simulink model "mMultiTorsionalCompliance"  (R2019b)
settings: Solver=ode4  StartTime=0.0  StopTime=1  FixedStep=.001  RelTol=1e-3
undefined symbols (not defined in the file): DiffAxleDamping, DiffAxleStiffness, DiffDriveshaftDamping, DiffDriveshaftStiffness
libraries: autolibsharedcoupling x6, autolibshareddiff x3, autolibpowerinfoutils x2, VsrLibCoupling x1
settings Model: Creator=9bt  LastModifiedBy=4qz

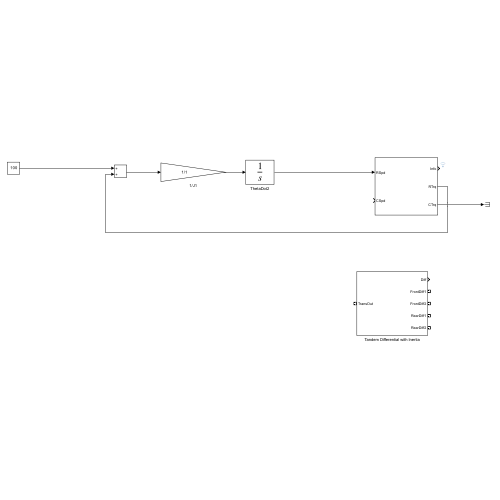
[thumbnail: Simulink's stored preview of the top-level diagram]
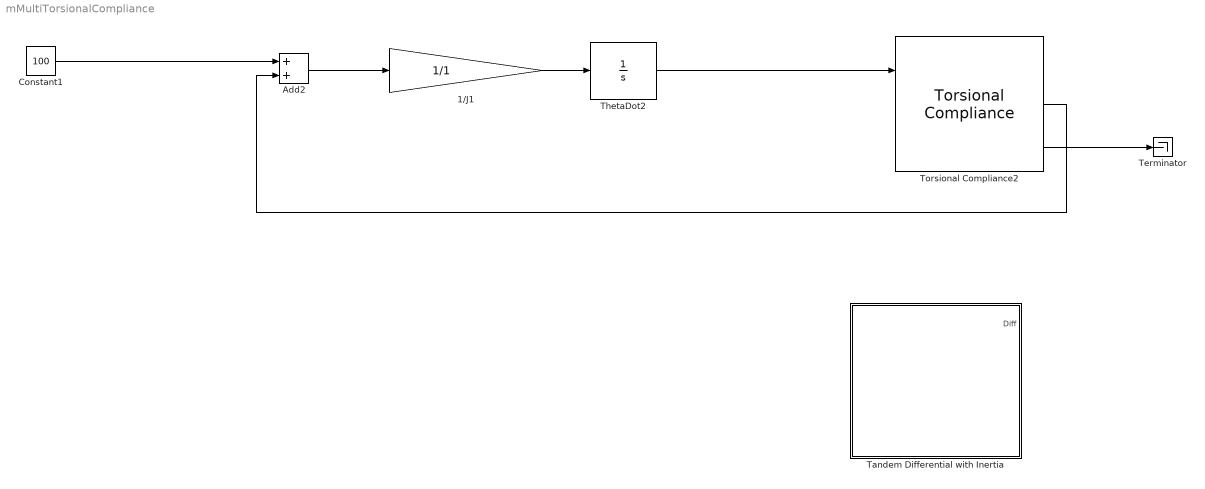
== system mMultiTorsionalCompliance ==
  1/J1 : Gain  Gain=1/1
  Add2 : Sum
  Constant1 : Constant  Value=100
  Tandem Differential with Inertia : Subsystem
  Terminator : Terminator
  ThetaDot2 : Integrator
  Torsional Compliance2 : VsrLibCoupling/Torsional Compliance  StiffnessCalcMethodPopup=Shaft dimensions and material properties  DampingCalcMethodPopup=Damping ratio  D_o=.066  D_i=0  L_shaft=.05  G=77e9  Jcalc=1  zeta=.5  wn=1693.7456  wd=1466.8267  k=2868774.14  b=1197.659  omega_c=500  theta_0=0  omega_0=0
  wires:
  ThetaDot2/1 -> Torsional Compliance2/1
  Add2/1 -> 1/J1/1
  Constant1/1 -> Add2/1
  1/J1/1 -> ThetaDot2/1
  Torsional Compliance2/2 -> Add2/2
  Torsional Compliance2/3 -> Terminator/1

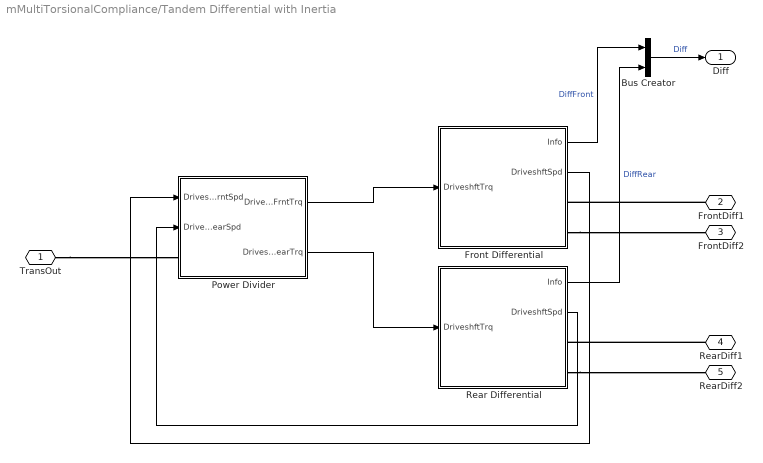
== system mMultiTorsionalCompliance/Tandem Differential with Inertia ==
  Bus Creator : BusCreator  Inputs=2
  Front Differential : Subsystem
  Power Divider : Subsystem
  Rear Differential : Subsystem
  TransOut : PMIOPort  Side=Left
  FrontDiff1 : PMIOPort  Port=2  Side=Right
  FrontDiff2 : PMIOPort  Port=3  Side=Right
  RearDiff1 : PMIOPort  Port=4  Side=Right
  RearDiff2 : PMIOPort  Port=5  Side=Right
  Diff : Outport
  wires:
  Front Differential/1(Info) -> Bus Creator/1  "DiffFront"
  Rear Differential/1(Info) -> Bus Creator/2  "DiffRear"
  Power Divider/2(DriveshftRearTrq) -> Rear Differential/1(DriveshftTrq)
  Power Divider/1(DriveshftFrntTrq) -> Front Differential/1(DriveshftTrq)
  Front Differential/2(DriveshftSpd) -> Power Divider/1(DriveshftFrntSpd)
  Bus Creator/1 -> Diff/1  "Diff"
  Rear Differential/2(DriveshftSpd) -> Power Divider/2(DriveshftRearSpd)
  connections:
  Rear Differential/RConn2 -- RearDiff2/RConn1
  RearDiff1/RConn1 -- Rear Differential/RConn1
  Front Differential/RConn2 -- FrontDiff2/RConn1
  TransOut/RConn1 -- Power Divider/LConn1
  FrontDiff1/RConn1 -- Front Differential/RConn1

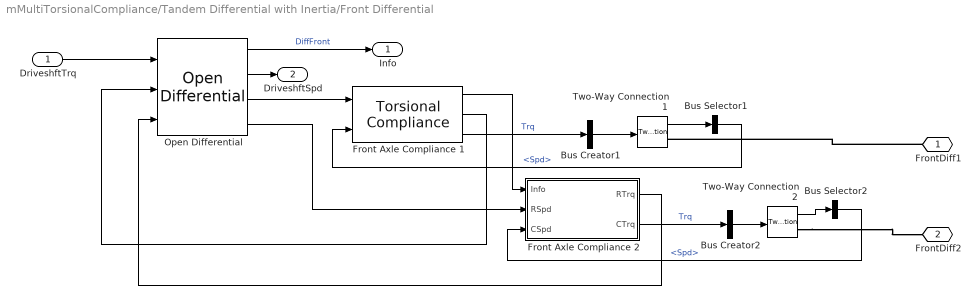
== system mMultiTorsionalCompliance/Tandem Differential with Inertia/Front Differential ==
  DriveshftTrq : Inport
  Bus Creator1 : BusCreator  Inputs=1
  Bus Creator2 : BusCreator  Inputs=1
  Bus Selector1 : BusSelector  OutputSignals=Spd
  Bus Selector2 : BusSelector  OutputSignals=Spd
  Front Axle Compliance 1 : autolibsharedcoupling/Torsional Compliance  port_config=Simulink  extInfo=on  k=DiffAxleStiffness  b=DiffAxleDamping  theta_o=0  domega_o=0  omega_c=DiffAxleCutoffFreq  blkID=0  aMode=1
  Front Axle Compliance 2 : Subsystem
  Open Differential : autolibshareddiff/Open Differential  DiffEffModelPopup=Constant  InterpMethod=Linear point-slope  extTamb=off  shaftSwitchMask=To the left of center-line  Ndiff=DiffFrontRatio  Jd=DiffFontCarrierInertia  bd=DiffFrontCarrierDamping  Jw1=DiffFrontAxleInertia  bw1=DiffFrontAxleDamping  Jw2=DiffFrontAxleInertia  bw2=DiffFrontAxleDamping  omegaw1o=0  omegaw2o=0  eta=DiffFrontEff  eta_tbl=reshape([0.64 0.76 0.8 0.81 0.83 0.84 0.84 0.56 0.73 0.78 0.8 0.83 0.84 0.84 0.54 0.71 0.77 0.8 0.82 0.84 0.84 0.53 0.71 0.77 0.8 0.83 0.84 0.84 0.51 0.71 0.77 0.8 0.83 0.84 0.85 0.52 0.7 0.77 0.8 0.83 0.84 0.85 0.51 0.71 0.76 0.79 0.83 0.84 0.85 0.5 0.69 0.76 0.79 0.82 0.84 0.85 0.45 0.68 0.75 0.78 0.82 0.84 0.85 0.43 0.67 0.74 0.78 0.81 0.83 0.84 0.38 0.63 0.71 0.75 0.8 0.82 0.83 0.81 0.86 0.88 0.89 0.89 0.89 0.9 0.77 0.85 0.87 0.88 0.89 0.9 0.9 0.72 0.82 0.86 0.87 0.88 0.89 0.9 0.68 0.8 0.84 0.86 0.88 0.89 0.89 0.67 0.8 0.84 0.86 0.88 0.89 0.9 0.67 0.8 0.84 0.86 0.88 0.89 0.9 0.65 0.8 0.84 0.86 0.88 0.89 0.9 0.64 0.79 0.83 0.86 0.88 0.89 0.9 0.63 0.78 0.83 0.86 0.88 0.89 0.9 0.59 0.76 0.82 0.85 0.87 0.89 0.9 0.53 0.73 0.8 0.83 0.86 0.88 0.89], 7, 11, 2)  Trq_bpts=[25, 50, 75, 100, 150, 200, 250]  omega_bpts=[52.4 78.5 105 131 157 183 209 262 314 419 524]  Temp_bpts=[290 358]  Tamb=297.15  maxAbsSpd=5e3  aMode=1
  Two-Way Connection1 : TwoWayConnection
  Two-Way Connection2 : TwoWayConnection
  FrontDiff1 : PMIOPort  Side=Right
  FrontDiff2 : PMIOPort  Port=2  Side=Right
  Info : Outport
  DriveshftSpd : Outport  Port=2
  wires:
  DriveshftTrq/1 -> Open Differential/1
  Open Differential/2 -> DriveshftSpd/1
  Open Differential/4 -> Front Axle Compliance 2/2(RSpd)
  Front Axle Compliance 1/3 -> Bus Creator1/1  "Trq"
  Front Axle Compliance 2/1(RTrq) -> Open Differential/3
  Open Differential/1 -> Info/1  "DiffFront"
  Bus Selector2/1 -> Front Axle Compliance 2/3(CSpd)  "<Spd>"
  Front Axle Compliance 2/2(CTrq) -> Bus Creator2/1  "Trq"
  Two-Way Connection2/1 -> Bus Selector2/1
  Bus Creator2/1 -> Two-Way Connection2/1
  Front Axle Compliance 1/2 -> Open Differential/2
  Open Differential/3 -> Front Axle Compliance 1/1
  Bus Creator1/1 -> Two-Way Connection1/1
  Front Axle Compliance 1/1 -> Front Axle Compliance 2/1(Info)
  Two-Way Connection1/1 -> Bus Selector1/1
  Bus Selector1/1 -> Front Axle Compliance 1/2  "<Spd>"
  connections:
  FrontDiff1/RConn1 -- Two-Way Connection1/RConn1
  Two-Way Connection2/RConn1 -- FrontDiff2/RConn1

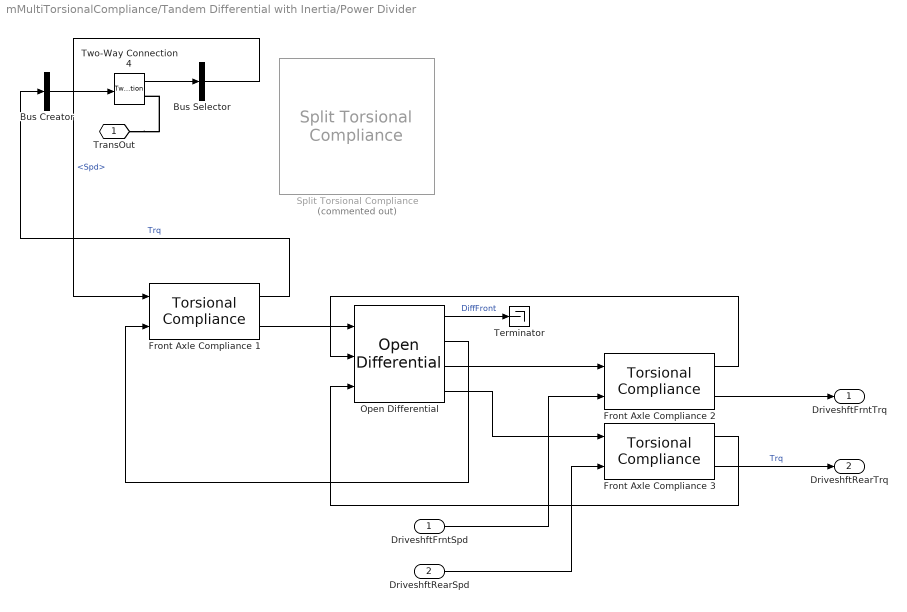
== system mMultiTorsionalCompliance/Tandem Differential with Inertia/Power Divider ==
  DriveshftFrntSpd : Inport
  DriveshftRearSpd : Inport  Port=2
  Bus Creator : BusCreator  Inputs=1
  Bus Selector : BusSelector  OutputSignals=Spd
  Front Axle Compliance 1 : autolibsharedcoupling/Torsional Compliance  port_config=Simulink  extInfo=off  k=DiffDriveshaftStiffness  b=DiffDriveshaftDamping  theta_o=0  domega_o=0  omega_c=DiffDriveshaftCuttoffFreq  blkID=0  aMode=1
  Front Axle Compliance 2 : autolibsharedcoupling/Torsional Compliance  port_config=Simulink  extInfo=off  k=DiffDriveshaftStiffness  b=DiffDriveshaftDamping  theta_o=0  domega_o=0  omega_c=DiffDriveshaftCuttoffFreq  blkID=0  aMode=1
  Front Axle Compliance 3 : autolibsharedcoupling/Torsional Compliance  port_config=Simulink  extInfo=off  k=DiffDriveshaftStiffness  b=DiffDriveshaftDamping  theta_o=0  domega_o=0  omega_c=DiffDriveshaftCuttoffFreq  blkID=0  aMode=1
  Open Differential : autolibshareddiff/Open Differential  DiffEffModelPopup=Constant  InterpMethod=Linear point-slope  extTamb=off  shaftSwitchMask=To the left of center-line  Ndiff=1  Jd=DiffFontCarrierInertia  bd=DiffFrontCarrierDamping  Jw1=DiffFrontAxleInertia  bw1=DiffFrontAxleDamping  Jw2=DiffFrontAxleInertia  bw2=DiffFrontAxleDamping  omegaw1o=0  omegaw2o=0  eta=DiffFrontEff  eta_tbl=reshape([0.64 0.76 0.8 0.81 0.83 0.84 0.84 0.56 0.73 0.78 0.8 0.83 0.84 0.84 0.54 0.71 0.77 0.8 0.82 0.84 0.84 0.53 0.71 0.77 0.8 0.83 0.84 0.84 0.51 0.71 0.77 0.8 0.83 0.84 0.85 0.52 0.7 0.77 0.8 0.83 0.84 0.85 0.51 0.71 0.76 0.79 0.83 0.84 0.85 0.5 0.69 0.76 0.79 0.82 0.84 0.85 0.45 0.68 0.75 0.78 0.82 0.84 0.85 0.43 0.67 0.74 0.78 0.81 0.83 0.84 0.38 0.63 0.71 0.75 0.8 0.82 0.83 0.81 0.86 0.88 0.89 0.89 0.89 0.9 0.77 0.85 0.87 0.88 0.89 0.9 0.9 0.72 0.82 0.86 0.87 0.88 0.89 0.9 0.68 0.8 0.84 0.86 0.88 0.89 0.89 0.67 0.8 0.84 0.86 0.88 0.89 0.9 0.67 0.8 0.84 0.86 0.88 0.89 0.9 0.65 0.8 0.84 0.86 0.88 0.89 0.9 0.64 0.79 0.83 0.86 0.88 0.89 0.9 0.63 0.78 0.83 0.86 0.88 0.89 0.9 0.59 0.76 0.82 0.85 0.87 0.89 0.9 0.53 0.73 0.8 0.83 0.86 0.88 0.89], 7, 11, 2)  Trq_bpts=[25, 50, 75, 100, 150, 200, 250]  omega_bpts=[52.4 78.5 105 131 157 183 209 262 314 419 524]  Temp_bpts=[290 358]  Tamb=297.15  maxAbsSpd=5e3  aMode=1
  Split Torsional Compliance : autolibsharedcoupling/Split Torsional Compliance  Commented=on  port_config=Simulink  cplrMode=Shaft split  extInfo=off  k1=DiffDriveshaftStiffness  b1=DiffDriveshaftDamping  omega1_c=DiffDriveshaftCuttoffFreq  theta1_o=0  domega1_o=0  k2=DiffDriveshaftStiffness  b2=DiffDriveshaftDamping  omega2_c=DiffDriveshaftCuttoffFreq  theta2_o=0  domega2_o=0  blkID=0  aMode=1
  Terminator : Terminator
  Two-Way Connection4 : TwoWayConnection
  TransOut : PMIOPort  Side=Left
  DriveshftFrntTrq : Outport
  DriveshftRearTrq : Outport  Port=2
  wires:
  Front Axle Compliance 2/2 -> DriveshftFrntTrq/1
  Bus Selector/1 -> Front Axle Compliance 1/1  "<Spd>"
  DriveshftRearSpd/1 -> Front Axle Compliance 3/2
  Front Axle Compliance 1/1 -> Bus Creator/1  "Trq"
  Two-Way Connection4/1 -> Bus Selector/1
  Bus Creator/1 -> Two-Way Connection4/1
  DriveshftFrntSpd/1 -> Front Axle Compliance 2/2
  Front Axle Compliance 1/2 -> Open Differential/1
  Open Differential/2 -> Front Axle Compliance 1/2
  Open Differential/1 -> Terminator/1  "DiffFront"
  Open Differential/4 -> Front Axle Compliance 3/1
  Open Differential/3 -> Front Axle Compliance 2/1
  Front Axle Compliance 3/2 -> DriveshftRearTrq/1  "Trq"
  Front Axle Compliance 3/1 -> Open Differential/3
  Front Axle Compliance 2/1 -> Open Differential/2
  connections:
  TransOut/RConn1 -- Two-Way Connection4/RConn1

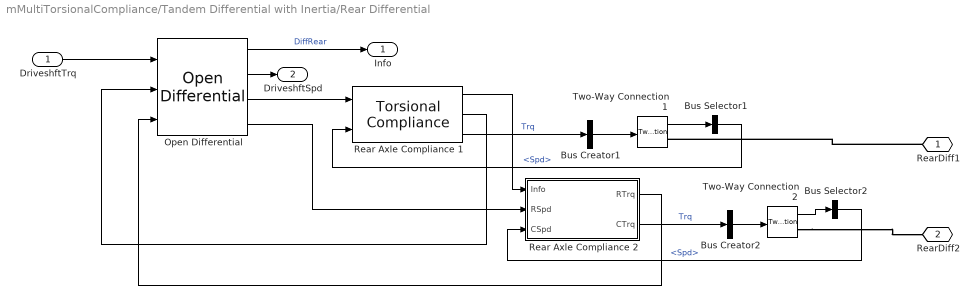
== system mMultiTorsionalCompliance/Tandem Differential with Inertia/Rear Differential ==
  DriveshftTrq : Inport
  Bus Creator1 : BusCreator  Inputs=1
  Bus Creator2 : BusCreator  Inputs=1
  Bus Selector1 : BusSelector  OutputSignals=Spd
  Bus Selector2 : BusSelector  OutputSignals=Spd
  Open Differential : autolibshareddiff/Open Differential  DiffEffModelPopup=Constant  InterpMethod=Linear point-slope  extTamb=off  shaftSwitchMask=To the left of center-line  Ndiff=DiffRearRatio  Jd=DiffRearCarrierInertia  bd=DiffRearCarrierDamping  Jw1=DiffRearAxleInertia  bw1=DiffRearAxleDamping  Jw2=DiffRearAxleInertia  bw2=DiffRearAxleDamping  omegaw1o=0  omegaw2o=0  eta=DiffRearEff  eta_tbl=reshape([0.64 0.76 0.8 0.81 0.83 0.84 0.84 0.56 0.73 0.78 0.8 0.83 0.84 0.84 0.54 0.71 0.77 0.8 0.82 0.84 0.84 0.53 0.71 0.77 0.8 0.83 0.84 0.84 0.51 0.71 0.77 0.8 0.83 0.84 0.85 0.52 0.7 0.77 0.8 0.83 0.84 0.85 0.51 0.71 0.76 0.79 0.83 0.84 0.85 0.5 0.69 0.76 0.79 0.82 0.84 0.85 0.45 0.68 0.75 0.78 0.82 0.84 0.85 0.43 0.67 0.74 0.78 0.81 0.83 0.84 0.38 0.63 0.71 0.75 0.8 0.82 0.83 0.81 0.86 0.88 0.89 0.89 0.89 0.9 0.77 0.85 0.87 0.88 0.89 0.9 0.9 0.72 0.82 0.86 0.87 0.88 0.89 0.9 0.68 0.8 0.84 0.86 0.88 0.89 0.89 0.67 0.8 0.84 0.86 0.88 0.89 0.9 0.67 0.8 0.84 0.86 0.88 0.89 0.9 0.65 0.8 0.84 0.86 0.88 0.89 0.9 0.64 0.79 0.83 0.86 0.88 0.89 0.9 0.63 0.78 0.83 0.86 0.88 0.89 0.9 0.59 0.76 0.82 0.85 0.87 0.89 0.9 0.53 0.73 0.8 0.83 0.86 0.88 0.89], 7, 11, 2)  Trq_bpts=[25, 50, 75, 100, 150, 200, 250]  omega_bpts=[52.4 78.5 105 131 157 183 209 262 314 419 524]  Temp_bpts=[290 358]  Tamb=297.15  maxAbsSpd=5e3  aMode=1
  Rear Axle Compliance 1 : autolibsharedcoupling/Torsional Compliance  port_config=Simulink  extInfo=on  k=DiffAxleStiffness  b=DiffAxleDamping  theta_o=0  domega_o=0  omega_c=DiffAxleCutoffFreq  blkID=0  aMode=1
  Rear Axle Compliance 2 : Subsystem
  Two-Way Connection1 : TwoWayConnection
  Two-Way Connection2 : TwoWayConnection
  RearDiff1 : PMIOPort  Side=Right
  RearDiff2 : PMIOPort  Port=2  Side=Right
  Info : Outport
  DriveshftSpd : Outport  Port=2
  wires:
  Open Differential/1 -> Info/1  "DiffRear"
  Bus Selector1/1 -> Rear Axle Compliance 1/2  "<Spd>"
  Two-Way Connection1/1 -> Bus Selector1/1
  Rear Axle Compliance 1/1 -> Rear Axle Compliance 2/1(Info)
  Bus Creator1/1 -> Two-Way Connection1/1
  Open Differential/3 -> Rear Axle Compliance 1/1
  Rear Axle Compliance 1/2 -> Open Differential/2
  Bus Creator2/1 -> Two-Way Connection2/1
  Two-Way Connection2/1 -> Bus Selector2/1
  Rear Axle Compliance 2/2(CTrq) -> Bus Creator2/1  "Trq"
  Bus Selector2/1 -> Rear Axle Compliance 2/3(CSpd)  "<Spd>"
  Rear Axle Compliance 2/1(RTrq) -> Open Differential/3
  Rear Axle Compliance 1/3 -> Bus Creator1/1  "Trq"
  Open Differential/4 -> Rear Axle Compliance 2/2(RSpd)
  Open Differential/2 -> DriveshftSpd/1
  DriveshftTrq/1 -> Open Differential/1
  connections:
  Two-Way Connection2/RConn1 -- RearDiff2/RConn1
  RearDiff1/RConn1 -- Two-Way Connection1/RConn1

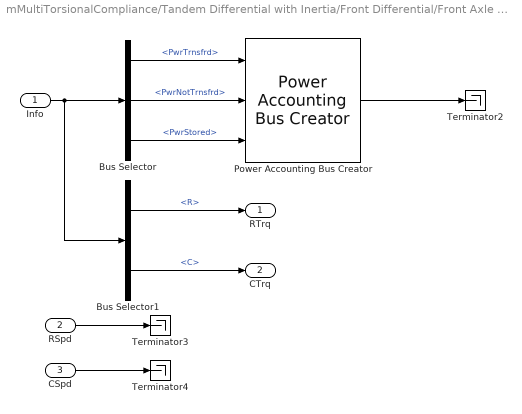
== system mMultiTorsionalCompliance/Tandem Differential with Inertia/Front Differential/Front Axle Compliance 2 ==
  Info : Inport
  RSpd : Inport  Port=2
  CSpd : Inport  Port=3
  Bus Selector : BusSelector  OutputSignals=PwrInfo.PwrTrnsfrd,PwrInfo.PwrNotTrnsfrd,PwrInfo.PwrStored
  Bus Selector1 : BusSelector  OutputSignals=Trq.R,Trq.C
  Power Accounting Bus Creator : autolibpowerinfoutils/Power Accounting Bus Creator  AssctBlkSelPopup=Parent  RefBlkName='libraryname/blkname'  PwrTrnsfrdCheckBox=on  PwrNotTrnsfrdCheckBox=on  PwrStoredCheckBox=on  aMode=aMode
  Terminator2 : Terminator
  Terminator3 : Terminator
  Terminator4 : Terminator
  RTrq : Outport
  CTrq : Outport  Port=2
  wires:
  RSpd/1 -> Terminator3/1
  CSpd/1 -> Terminator4/1
  Bus Selector/3 -> Power Accounting Bus Creator/3  "<PwrStored>"
  Bus Selector/2 -> Power Accounting Bus Creator/2  "<PwrNotTrnsfrd>"
  Bus Selector/1 -> Power Accounting Bus Creator/1  "<PwrTrnsfrd>"
  Power Accounting Bus Creator/1 -> Terminator2/1
  Bus Selector1/2 -> CTrq/1  "<C>"
  Bus Selector1/1 -> RTrq/1  "<R>"
  Info/1 -> Bus Selector/1, Bus Selector1/1

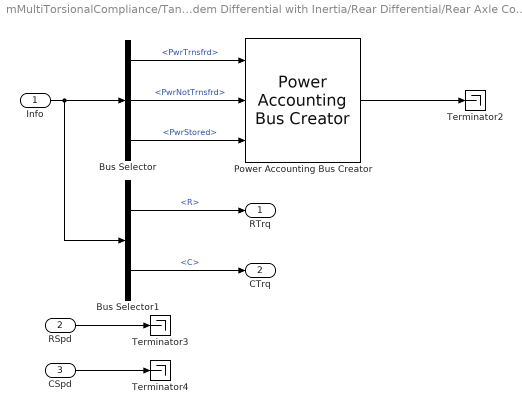
== system mMultiTorsionalCompliance/Tandem Differential with Inertia/Rear Differential/Rear Axle Compliance 2 ==
  Info : Inport
  RSpd : Inport  Port=2
  CSpd : Inport  Port=3
  Bus Selector : BusSelector  OutputSignals=PwrInfo.PwrTrnsfrd,PwrInfo.PwrNotTrnsfrd,PwrInfo.PwrStored
  Bus Selector1 : BusSelector  OutputSignals=Trq.R,Trq.C
  Power Accounting Bus Creator : autolibpowerinfoutils/Power Accounting Bus Creator  AssctBlkSelPopup=Parent  RefBlkName='libraryname/blkname'  PwrTrnsfrdCheckBox=on  PwrNotTrnsfrdCheckBox=on  PwrStoredCheckBox=on  aMode=aMode
  Terminator2 : Terminator
  Terminator3 : Terminator
  Terminator4 : Terminator
  RTrq : Outport
  CTrq : Outport  Port=2
  wires:
  Info/1 -> Bus Selector1/1, Bus Selector/1
  Bus Selector1/1 -> RTrq/1  "<R>"
  Bus Selector1/2 -> CTrq/1  "<C>"
  Power Accounting Bus Creator/1 -> Terminator2/1
  Bus Selector/1 -> Power Accounting Bus Creator/1  "<PwrTrnsfrd>"
  Bus Selector/2 -> Power Accounting Bus Creator/2  "<PwrNotTrnsfrd>"
  Bus Selector/3 -> Power Accounting Bus Creator/3  "<PwrStored>"
  CSpd/1 -> Terminator4/1
  RSpd/1 -> Terminator3/1
